simulink model "Yolo"  (R2024a)
settings: Solver=VariableStepAuto  StartTime=0.0  StopTime=inf  RelTol=1e-3
undefined symbols (not defined in the file): Angle, Axis, gray
libraries: robotcorelib x4, eeGeneralControl x2
settings Model: Creator=user  LastModifiedBy=quentinlandon

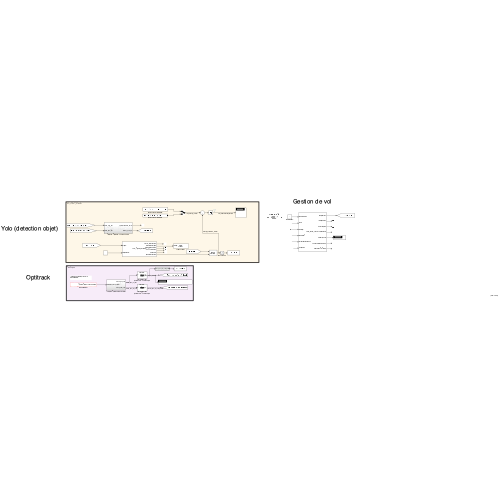
[thumbnail: Simulink's stored preview of the top-level diagram]
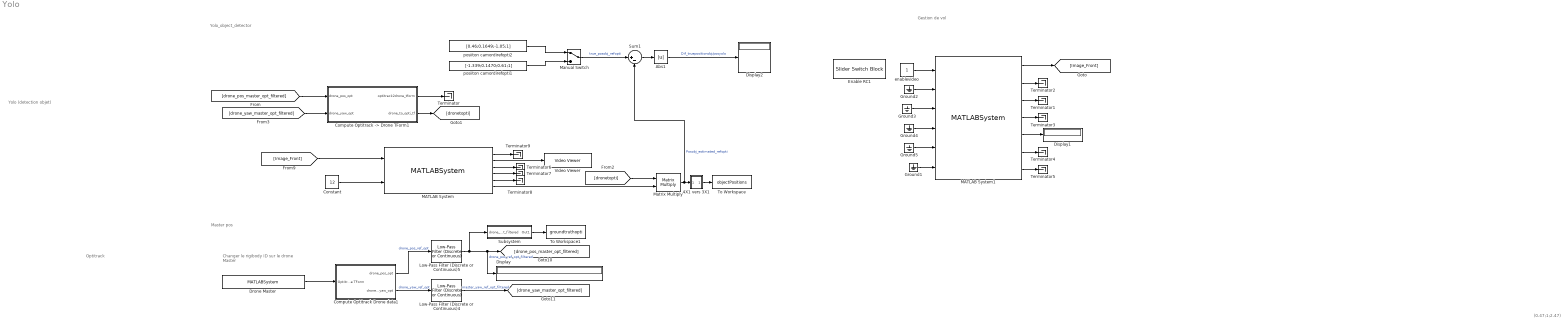
== system Yolo ==
  note: Yolo_object_detector
  note: Changer le rigibody ID sur le drone Master
  note: Master pos
  note: (0.47;1;2.47)
  note: Gestion de vol
  note: Yolo (detection objet)
  note: Optitrack
  4X1 vers 3X1 : Subsystem
  Abs1 : Abs  SaturateOnIntegerOverflow=off
  "Compute Optitrack -> Drone TForm1" : Subsystem
  Compute Optitrack Drone data1 : Subsystem
  Constant : Constant  Value=12
  Display : Display
  Display1 : Display
  Display2 : Display
  Drone Master : MATLABSystem  System=OptilinkSystem  HostIP=10.147.125.15  ClientIP=10.147.125.15  RigidbodyID=2  SimulateUsing=Interpreted execution
      mask Type: OptilinkSystem
      mask Display:
      | disp('OptilinkSystem');
      | port_label('output',1,'Drones data');
  Enable RC1 : SliderSwitchBlock
      settings: Values={{'Off', 'On'}, [0 1]}
  Ground{1..5} (5 alike) : Ground
  Low-Pass Filter (Discrete or Continuous)4 : eeGeneralControl/Low-Pass Filter (Discrete or Continuous)  K=1  T=1.5  B=inf  A=-inf  init_option=Inherited from block input  x0=0  Ts=-1
  Low-Pass Filter (Discrete or Continuous)5 : eeGeneralControl/Low-Pass Filter (Discrete or Continuous)  K=1  T=1.5  B=inf  A=-inf  init_option=Inherited from block input  x0=0  Ts=-1
  MATLAB System : MATLABSystem  System=Yolo_Object_Detector  SimulateUsing=Interpreted execution
      mask Type: Yolo_Object_Detector
      mask Display:
      | disp('Yolo_Object_Detector');
      | port_label('input',1,'Image');
      | port_label('input',2,'degreecam');
      | port_label('output',1,'Tform_camtodrone');
      | port_label('output',2,'AnnotatedImage');
      | port_label('output',3,'BBoxDimensions');
      | port_label('output',4,'CamCoordinates');
      | port_label('output',5,'posecam');
      | port_label('output',6,'posecamtodrone');
  MATLAB System1 : MATLABSystem  System=Tello_drone_control  droneIP=127.0.0.1  SimulateUsing=Interpreted execution
      mask Type: Tello_drone_control
      mask Display:
      | disp('Tello_drone_control');
      | port_label('input',1,'enableVideo');
      | port_label('input',2,'tkoff');
      | port_label('input',3,'landing');
      | port_label('input',4,'enableRC');
      | port_label('input',5,'cmdVideoDirection');
      | port_label('input',6,'rcspeeds');
      | port_label('output',1,'imageFront');
      | port_label('output',2,'imageDown');
      | port_label('output',3,'Eulerangles');
      | port_label('output',4,'speedXYZ');
      | port_label('output',5,'batteryLevel');
      | port_label('output',6,'currentVideoDirection');
      | port_label('output',7,'hasTakenOffStatus');
  Manual Switch : ManualSwitch
  Matrix Multiply : Product  Multiplication=Matrix(*)
  Subsystem : Subsystem
  Sum1 : Sum  Inputs=|+-
  Terminator{,1..9} (10 alike) : Terminator
  To Workspace : ToWorkspace  VariableName=objectPositions  SampleTime=-1
  To Workspace1 : ToWorkspace  VariableName=groundtruthopti  SampleTime=-1
  Video Viewer : VideoViewer  colormapValue=gray(256)  FigPos=[-1470 1113 894 700]
  enablevideo : Constant
  posiiton camordirefopti1 : Constant  Value=[-1.339;0.1470;0.61;1]
  posiiton camordirefopti2 : Constant  Value=[0.46;0.1649;-1.05;1]
  wires:
  MATLAB System/2 -> Video Viewer/1
  [Image_Front] -> MATLAB System/1
  Low-Pass Filter (Discrete or Continuous)4/1 -> [drone_yaw_master_opt_filtered]  "master_yaw_ref_opt_filtered"
  Low-Pass Filter (Discrete or Continuous)5/1 -> Display/1, [drone_pos_master_opt_filtered], Subsystem/1(drone_pos_ref_opt_filtered)  "drone_pos_ref_opt_filtered"
  Compute Optitrack Drone data1/2(drone_yaw_opt) -> Low-Pass Filter (Discrete or Continuous)4/1  "drone_yaw_ref_opt"
  Drone Master/1 -> Compute Optitrack Drone data1/1(Optitrack Drone TForm)
  Compute Optitrack Drone data1/1(drone_pos_opt) -> Low-Pass Filter (Discrete or Continuous)5/1  "drone_pos_ref_opt"
  enablevideo/1 -> MATLAB System1/1
  MATLAB System1/2 -> Terminator2/1
  MATLAB System1/3 -> Terminator1/1
  MATLAB System1/4 -> Terminator3/1
  Ground1/1 -> MATLAB System1/6
  Ground3/1 -> MATLAB System1/3
  MATLAB System1/5 -> Display1/1
  MATLAB System1/7 -> Terminator5/1
  Ground4/1 -> MATLAB System1/4
  Ground2/1 -> MATLAB System1/2
  MATLAB System1/6 -> Terminator4/1
  Ground5/1 -> MATLAB System1/5
  MATLAB System1/1 -> [Image_Front]
  [drone_pos_master_opt_filtered] -> "Compute Optitrack -> Drone TForm1"/1(drone_pos_opt)
  [drone_yaw_master_opt_filtered] -> "Compute Optitrack -> Drone TForm1"/2(drone_yaw_opt)
  "Compute Optitrack -> Drone TForm1"/1(optitrack2drone_tform) -> Terminator/1
  "Compute Optitrack -> Drone TForm1"/2(drone_to_opti_tf) -> [dronetopti]
  Sum1/1 -> Abs1/1
  Abs1/1 -> Display2/1  "Dif_truepositionobj/posyolo"
  MATLAB System/3 -> Terminator6/1
  MATLAB System/4 -> Terminator7/1
  MATLAB System/5 -> Terminator8/1
  MATLAB System/6 -> Matrix Multiply/2
  [dronetopti] -> Matrix Multiply/1
  Matrix Multiply/1 -> Sum1/2, 4X1 vers 3X1/1(In1)  "Posobj_estimated_refopti"
  Constant/1 -> MATLAB System/2
  posiiton camordirefopti2/1 -> Manual Switch/1
  posiiton camordirefopti1/1 -> Manual Switch/2
  Manual Switch/1 -> Sum1/1  "true_posobj_refopti"
  Subsystem/1(Out1) -> To Workspace1/1
  4X1 vers 3X1/1(Out1) -> To Workspace/1
  MATLAB System/1 -> Terminator9/1

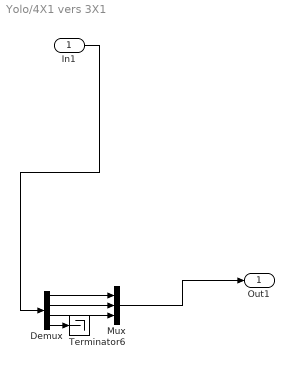
== system Yolo/4X1 vers 3X1 ==
  In1 : Inport
  Demux : Demux
  Mux : Mux  Inputs=3
  Terminator6 : Terminator
  Out1 : Outport
  wires:
  Mux/1 -> Out1/1
  Demux/2 -> Mux/2
  Demux/3 -> Mux/3
  Demux/4 -> Terminator6/1
  Demux/1 -> Mux/1
  In1/1 -> Demux/1

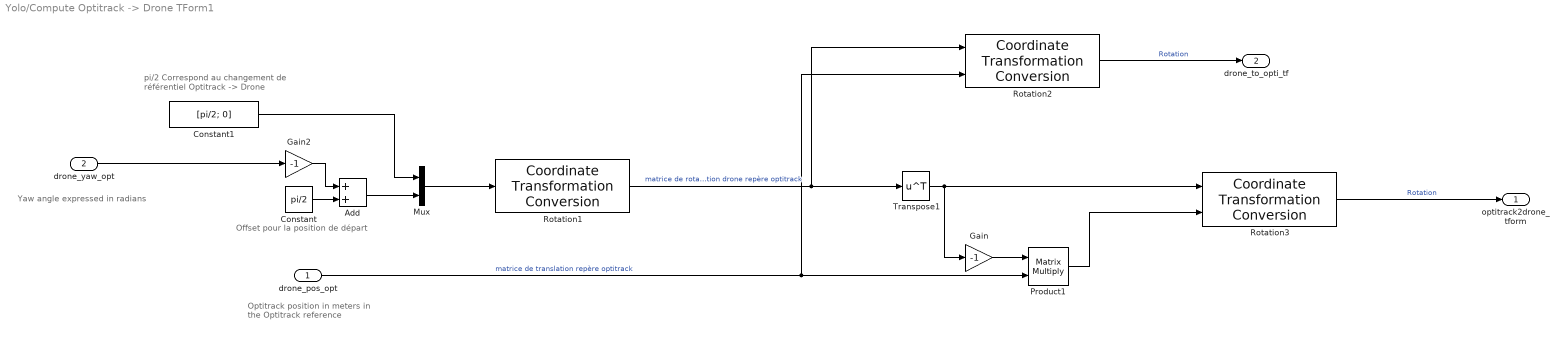
== system Yolo/Compute Optitrack -> Drone TForm1 ==
  note: Yaw angle expressed in radians
  note: Offset pour la position de départ
  note: pi/2 Correspond au changement de référentiel Optitrack -> Drone
  note: Optitrack position in meters
      | in the Optitrack reference
  drone_pos_opt : Inport
  drone_yaw_opt : Inport  Port=2
  Add : Sum
  Constant : Constant  Value=pi/2
  Constant1 : Constant  Value=[pi/2; 0]
  Gain : Gain  Gain=-1
  Gain2 : Gain  Gain=-1
  Mux : Mux  Inputs=2
  Product1 : Product  Multiplication=Matrix(*)
  Rotation1 : robotcorelib/Coordinate Transformation Conversion  InputRepresentation=Euler Angles  InputEulerSequence=XYZ  ShowTrVecInputPort=off  OutputRepresentation=Rotation Matrix  OutputEulerSequence=ZYX  ShowTrVecOutputPort=off  SimulateUsing=Code generation
      settings: LibrarySourceBlock=uavutilslib/Coordinate Transformation Conversion
  Rotation2 : robotcorelib/Coordinate Transformation Conversion  InputRepresentation=Rotation Matrix  InputEulerSequence=XYZ  ShowTrVecInputPort=on  OutputRepresentation=Homogeneous Transformation  OutputEulerSequence=ZYX  ShowTrVecOutputPort=off  SimulateUsing=Code generation
      settings: LibrarySourceBlock=uavutilslib/Coordinate Transformation Conversion
  Rotation3 : robotcorelib/Coordinate Transformation Conversion  InputRepresentation=Rotation Matrix  InputEulerSequence=XYZ  ShowTrVecInputPort=on  OutputRepresentation=Homogeneous Transformation  OutputEulerSequence=ZYX  ShowTrVecOutputPort=off  SimulateUsing=Code generation
      settings: LibrarySourceBlock=uavutilslib/Coordinate Transformation Conversion
  Transpose1 : Math  Operator=transpose
  optitrack2drone_tform : Outport
  drone_to_opti_tf : Outport  Port=2
  wires:
  Add/1 -> Mux/2
  Transpose1/1 -> Rotation3/1, Gain/1
  Constant/1 -> Add/2
  Gain2/1 -> Add/1
  Product1/1 -> Rotation3/2
  Constant1/1 -> Mux/1
  Rotation1/1 -> Rotation2/1, Transpose1/1  "matrice de rotation drone repère optitrack"
  Gain/1 -> Product1/1
  Mux/1 -> Rotation1/1
  drone_pos_opt/1 -> Rotation2/2, Product1/2  "matrice de translation repère optitrack"
  drone_yaw_opt/1 -> Gain2/1
  Rotation3/1 -> optitrack2drone_tform/1  "Rotation"
  Rotation2/1 -> drone_to_opti_tf/1  "Rotation"

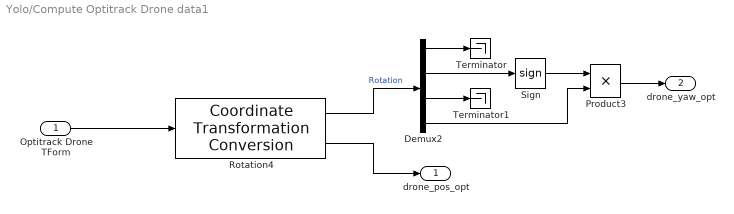
== system Yolo/Compute Optitrack Drone data1 ==
  Optitrack Drone TForm : Inport
  Demux2 : Demux
  Product3 : Product
  Rotation4 : robotcorelib/Coordinate Transformation Conversion  InputRepresentation=Homogeneous Transformation  InputEulerSequence=XYZ  ShowTrVecInputPort=on  OutputRepresentation=Axis-Angle  OutputEulerSequence=XYZ  ShowTrVecOutputPort=on  SimulateUsing=Code generation
      settings: LibrarySourceBlock=uavutilslib/Coordinate Transformation Conversion
  Sign : Signum
  Terminator : Terminator
  Terminator1 : Terminator
  drone_pos_opt : Outport
  drone_yaw_opt : Outport  Port=2
  wires:
  Rotation4/2 -> drone_pos_opt/1
  Demux2/4 -> Product3/2
  Rotation4/1 -> Demux2/1  "Rotation"
  Sign/1 -> Product3/1
  Demux2/2 -> Sign/1
  Product3/1 -> drone_yaw_opt/1
  Optitrack Drone TForm/1 -> Rotation4/1
  Demux2/3 -> Terminator1/1
  Demux2/1 -> Terminator/1

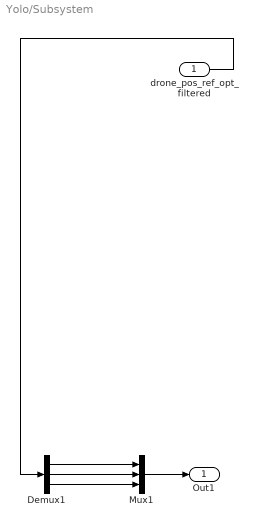
== system Yolo/Subsystem ==
  drone_pos_ref_opt_filtered : Inport
  Demux1 : Demux  Outputs=3
  Mux1 : Mux  Inputs=3
  Out1 : Outport
  wires:
  drone_pos_ref_opt_filtered/1 -> Demux1/1
  Mux1/1 -> Out1/1
  Demux1/3 -> Mux1/3
  Demux1/1 -> Mux1/1
  Demux1/2 -> Mux1/2
